simulink model "DSBFC"  (R2023b)
settings: Solver=VariableStepAuto  StartTime=0.0  StopTime=10  RelTol=1e-3
libraries: simulink x1
settings Model: Creator=HP  LastModifiedBy=HP

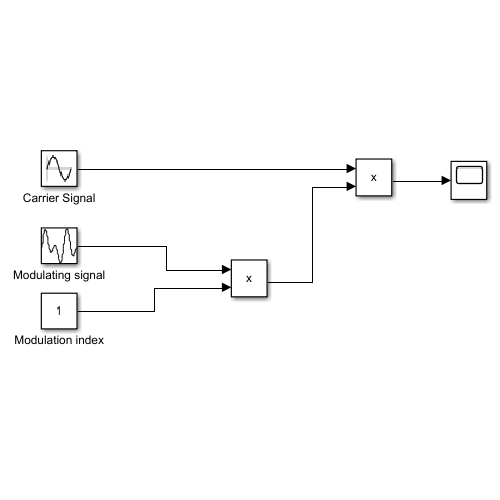
[thumbnail: Simulink's stored preview of the top-level diagram]
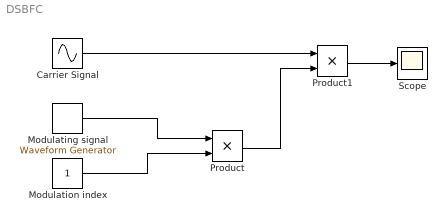
== system DSBFC ==
  Carrier Signal : Sin  Amplitude=5  Frequency=50  SampleTime=0
  Modulating signal : simulink/Sources/Waveform Generator  OutMin=[]  OutMax=[]  OutDataTypeStr=Inherit: Inherit via back propagation  SelectedSignal=1  Signals=sin(5,5,1)  BlockNames=MultiportSwitch_1e26bf96150c493  SampleTime=0.1
  Modulation index : Constant
  Product : Product
  Product1 : Product
  Scope : Scope
  wires:
  Carrier Signal/1 -> Product1/1
  Modulating signal/1 -> Product/1
  Modulation index/1 -> Product/2
  Product/1 -> Product1/2
  Product1/1 -> Scope/1
